simulink model "task4_lab2"  (R2020b)
settings: Solver=VariableStepAuto  StartTime=0.0  StopTime=0.3  RelTol=1e-3  EnableMultiTasking=on
settings Model: Creator=JackShen  LastModifiedBy=mluser
settings DataIOCC: LimitDataPoints=on  ReturnWorkspaceOutputs=off
settings OptimizationCC: LifeSpan=inf
settings DebuggingCC: AllowSymbolicDim=off  SFUnexpectedBacktrackingDiag=warning  SFNoUnconditionalDefaultTransitionDiag=warning  SFExecutionAtInitializationDiag=none  ArithmeticOperatorsInVariantConditions=warning
settings ModelReferenceCC: PropagateSignalLabelsOutOfModel=off
settings SFSimCC: SimUseLocalCustomCode=off  CustomCodeUndefinedFunction=UseInterfaceOnly
settings RTWCC: RTWUseLocalCustomCode=off
settings CodeAppCC: StateflowObjectComments=on
settings GRTTargetCC: TargetLangStandard=C89/C90 (ANSI)
settings ConfigComp: CovMetricSettings=dw  CovSaveCumulativeToWorkspaceVar=on  CovSaveSingleToWorkspaceVar=on  CovExternalEMLEnable=off

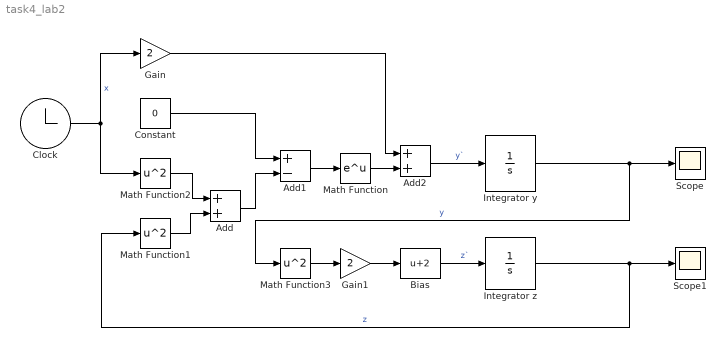
== system task4_lab2 ==
  Add : Sum
  Add1 : Sum  Inputs=+-
  Add2 : Sum
  Bias : Bias  Bias=2
  Clock : Clock
  Constant : Constant  Value=0
  Gain : Gain  Gain=2
  Gain1 : Gain  Gain=2
  Integrator y : Integrator  InitialCondition=0.5
  Integrator z : Integrator  InitialCondition=1
  Math Function : Math  SignedPower=on  SaturateOnIntegerOverflow=on
  Math Function1 : Math  Operator=square  SignedPower=on  SaturateOnIntegerOverflow=on
  Math Function2 : Math  Operator=square  SignedPower=on  SaturateOnIntegerOverflow=on
  Math Function3 : Math  Operator=square  SignedPower=on  SaturateOnIntegerOverflow=on
  Scope : Scope
  Scope1 : Scope
  wires:
  Add2/1 -> Integrator y/1  "y`"
  Bias/1 -> Integrator z/1  "z`"
  Math Function1/1 -> Add/2
  Math Function2/1 -> Add/1
  Constant/1 -> Add1/1
  Add/1 -> Add1/2
  Add1/1 -> Math Function/1
  Math Function/1 -> Add2/2
  Gain/1 -> Add2/1
  Math Function3/1 -> Gain1/1
  Gain1/1 -> Bias/1
  Clock/1 -> Math Function2/1, Gain/1  "x"
  Integrator z/1 -> Math Function1/1, Scope1/1  "z"
  Integrator y/1 -> Scope/1, Math Function3/1  "y"
